simulink model "series_blance_leg"  (R2022b)
settings: Solver=ode45  StartTime=0.0  StopTime=10  MaxStep=0.2  RelTol=1e-3
values from neighbouring files (symbols this model uses):
  a11 = polyfit(leg,k11,3)    [series_get_k.m]
  a12 = polyfit(leg,k12,3)    [series_get_k.m]
  a13 = polyfit(leg,k13,3)    [series_get_k.m]
  a14 = polyfit(leg,k14,3)    [series_get_k.m]
  a15 = polyfit(leg,k15,3)    [series_get_k.m]
  a16 = polyfit(leg,k16,3)    [series_get_k.m]
  a21 = polyfit(leg,k21,3)    [series_get_k.m]
  a22 = polyfit(leg,k22,3)    [series_get_k.m]
  a23 = polyfit(leg,k23,3)    [series_get_k.m]
  a24 = polyfit(leg,k24,3)    [series_get_k.m]
  a25 = polyfit(leg,k25,3)    [series_get_k.m]
  a26 = polyfit(leg,k26,3)    [series_get_k.m]
  N = NM + mp*diff(x + L*sin(theta),t,2)    [series_get_k_length.m]
undefined symbols (not defined in the file or in its folder): X, Y, Z
libraries: sm_lib x60, nesl_utility x20, matrix_library x8, slpidlib x2, cstblocks x2
(part 3 of 3)

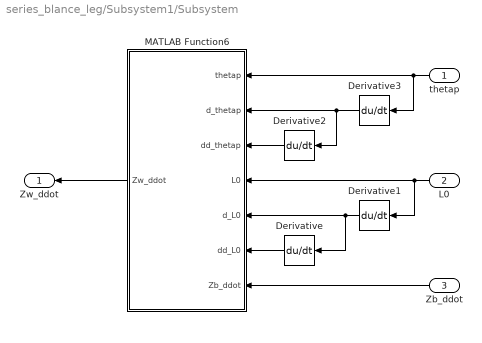
== system series_blance_leg/Subsystem1/Subsystem ==
  thetap : Inport
  L0 : Inport  Port=2
  Zb_ddot : Inport  Port=3
  Derivative{,1..3} (4 alike) : Derivative
  MATLAB Function6 : MATLAB Function  TreatAsAtomicUnit=on
  Zw_ddot : Outport
  wires:
  thetap/1 -> MATLAB Function6/1(thetap), Derivative3/1
  L0/1 -> Derivative1/1, MATLAB Function6/4(L0)
  Derivative1/1 -> Derivative/1, MATLAB Function6/5(d_L0)
  Derivative2/1 -> MATLAB Function6/3(dd_thetap)
  Derivative3/1 -> Derivative2/1, MATLAB Function6/2(d_thetap)
  Derivative/1 -> MATLAB Function6/6(dd_L0)
  Zb_ddot/1 -> MATLAB Function6/7(Zb_ddot)
  MATLAB Function6/1(Zw_ddot) -> Zw_ddot/1

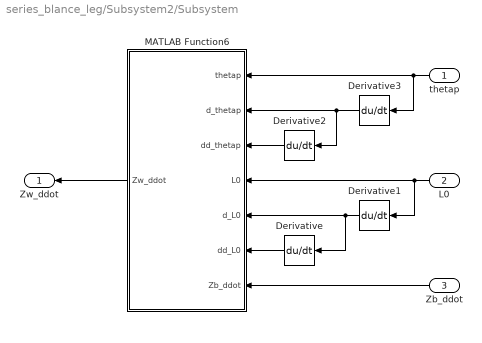
== system series_blance_leg/Subsystem2/Subsystem ==
  thetap : Inport
  L0 : Inport  Port=2
  Zb_ddot : Inport  Port=3
  Derivative{,1..3} (4 alike) : Derivative
  MATLAB Function6 : MATLAB Function  TreatAsAtomicUnit=on
  Zw_ddot : Outport
  wires:
  thetap/1 -> MATLAB Function6/1(thetap), Derivative3/1
  L0/1 -> Derivative1/1, MATLAB Function6/4(L0)
  Derivative1/1 -> Derivative/1, MATLAB Function6/5(d_L0)
  Derivative2/1 -> MATLAB Function6/3(dd_thetap)
  Derivative3/1 -> Derivative2/1, MATLAB Function6/2(d_thetap)
  Derivative/1 -> MATLAB Function6/6(dd_L0)
  Zb_ddot/1 -> MATLAB Function6/7(Zb_ddot)
  MATLAB Function6/1(Zw_ddot) -> Zw_ddot/1

== matlab function series_blance_leg/control/MATLAB Function8 ==
  data: d_phi0 output; theta1 input; theta2 input; d_theta1 input; d_theta2 input
function d_phi0 = D_PHI0(theta1,theta2,d_theta1,d_theta2)
   
    l1=0.3;
    l2=0.3;

    d_phi0 = (d_theta1*l1*(l1 + l2*cos(theta1 - theta2)))/(l1^2 + 2*cos(theta1 - theta2)*l1*l2 + l2^2) + (d_theta2*l2*(l2 + l1*cos(theta1 - theta2)))/(l1^2 + 2*cos(theta1 - theta2)*l1*l2 + l2^2);
 
    
end
    % jacobian函数无法在simulink中使用，故直接使用jacobian函数的最终结果

== matlab function series_blance_leg/calc/MATLAB Function6 ==
  data: k output; a input; length input
function k = get_K(a,length)
   k = polyval(a,length);  
end

== matlab function series_blance_leg/calc/MATLAB Function10 ==
  data: k output; a input; length input
function k = get_K(a,length)
   k = polyval(a,length);  
end

== matlab function series_blance_leg/calc/MATLAB Function11 ==
  data: k output; a input; length input
function k = get_K(a,length)
   k = polyval(a,length);  
end

== matlab function series_blance_leg/calc/MATLAB Function12 ==
  data: k output; a input; length input
function k = get_K(a,length)
   k = polyval(a,length);  
end

== matlab function series_blance_leg/calc/MATLAB Function7 ==
  data: k output; a input; length input
function k = get_K(a,length)
   k = polyval(a,length);  
end

== matlab function series_blance_leg/calc/MATLAB Function8 ==
  data: k output; a input; length input
function k = get_K(a,length)
   k = polyval(a,length);  
end

== matlab function series_blance_leg/control1/MATLAB Function6 ==
  data: F0 input; T1 output; Tp input; theta1 input; theta2 input; T2 output
function [T1,T2] = VMC_calc(F0,Tp,theta1,theta2)
  
l1=0.3;
l2=0.3;
   
j11 = -(l1*l2*sin(theta1 - theta2))/(l1^2 + 2*cos(theta1 - theta2)*l1*l2 + l2^2)^(1/2);
j12 = (l1*l2*sin(theta1 - theta2))/(l1^2 + 2*cos(theta1 - theta2)*l1*l2 + l2^2)^(1/2);
j21 = (l1*(l1 + l2*cos(theta1 - theta2)))/(l1^2 + 2*cos(theta1 - theta2)*l1*l2 + l2^2);
j22 = (l2*(l2 + l1*cos(theta1 - theta2)))/(l1^2 + 2*cos(theta1 - theta2)*l1*l2 + l2^2);
J = [j11 j12; j21 j22];
F = [F0;Tp];
T = J' * F;
T1 = T(1,1);
T2 = T(2,1);

end

== matlab function series_blance_leg/calc/MATLAB Function9 ==
  data: k output; a input; length input
function k = get_K(a,length)
   k = polyval(a,length);  
end

== matlab function series_blance_leg/calc1/MATLAB Function1 ==
  data: k output; a input; length input
function k = get_K(a,length)
   k = polyval(a,length);  
end

== matlab function series_blance_leg/calc1/MATLAB Function10 ==
  data: k output; a input; length input
function k = get_K(a,length)
   k = polyval(a,length);  
end

== matlab function series_blance_leg/calc1/MATLAB Function11 ==
  data: k output; a input; length input
function k = get_K(a,length)
   k = polyval(a,length);  
end

== matlab function series_blance_leg/calc1/MATLAB Function12 ==
  data: k output; a input; length input
function k = get_K(a,length)
   k = polyval(a,length);  
end

== matlab function series_blance_leg/calc1/MATLAB Function2 ==
  data: k output; a input; length input
function k = get_K(a,length)
   k = polyval(a,length);  
end

== matlab function series_blance_leg/calc1/MATLAB Function3 ==
  data: k output; a input; length input
function k = get_K(a,length)
   k = polyval(a,length);  
end

== matlab function series_blance_leg/calc1/MATLAB Function4 ==
  data: k output; a input; length input
function k = get_K(a,length)
   k = polyval(a,length);  
end

== matlab function series_blance_leg/calc1/MATLAB Function5 ==
  data: k output; a input; length input
function k = get_K(a,length)
   k = polyval(a,length);  
end

== matlab function series_blance_leg/calc1/MATLAB Function6 ==
  data: k output; a input; length input
function k = get_K(a,length)
   k = polyval(a,length);  
end

== matlab function series_blance_leg/calc1/MATLAB Function7 ==
  data: k output; a input; length input
function k = get_K(a,length)
   k = polyval(a,length);  
end

== matlab function series_blance_leg/calc1/MATLAB Function8 ==
  data: k output; a input; length input
function k = get_K(a,length)
   k = polyval(a,length);  
end

== matlab function series_blance_leg/calc1/MATLAB Function9 ==
  data: k output; a input; length input
function k = get_K(a,length)
   k = polyval(a,length);  
end

== matlab function series_blance_leg/Subsystem1/MATLAB Function6 ==
  data: thetap input; zw_ddot input; F input; Fn output
function Fn = Fn_calc(thetap,zw_ddot,F)
    
  Mp=5.54; 
  Mw=1.18;
  g=9.8;
  Fn=F*cos(thetap)+Mp*g+Mw*zw_ddot;
end

== matlab function series_blance_leg/control1/MATLAB Function7 ==
  data: L0 output; theta1 input; theta2 input; phi0 output
function [L0,phi0] = L0_PHI0(theta1,theta2)

l1=0.3;
l2=0.3;

xc = l1*cos(theta1) + l2*cos(theta2);
yc = l1*sin(theta1) + l2*sin(theta2);
L0 = sqrt(xc^2+yc^2);
phi0 = atan2(yc,xc);
end

== matlab function series_blance_leg/Subsystem1/Subsystem/MATLAB Function6 ==
  data: thetap input; Zw_ddot output; d_thetap input; dd_thetap input; L0 input; d_L0 input; dd_L0 input; Zb_ddot input
function Zw_ddot = Zw_ddot_calc(thetap,d_thetap,dd_thetap,L0,d_L0,dd_L0,Zb_ddot)

   Zw_ddot=Zb_ddot-dd_L0*cos(thetap)+2*d_L0*d_thetap*sin(thetap)+L0*dd_thetap*sin(thetap)+L0*(d_thetap^2)*cos(thetap);
end

== matlab function series_blance_leg/Subsystem2/MATLAB Function6 ==
  data: thetap input; zw_ddot input; F input; Fn output
function Fn = Fn_calc(thetap,zw_ddot,F)
    
  Mp=5.54; 
  Mw=1.18;
  g=9.8;
  Fn=F*cos(thetap)+Mp*g+Mw*zw_ddot;
end

== matlab function series_blance_leg/Subsystem2/Subsystem/MATLAB Function6 ==
  data: thetap input; Zw_ddot output; d_thetap input; dd_thetap input; L0 input; d_L0 input; dd_L0 input; Zb_ddot input
function Zw_ddot = Zw_ddot_calc(thetap,d_thetap,dd_thetap,L0,d_L0,dd_L0,Zb_ddot)

   Zw_ddot=Zb_ddot-dd_L0*cos(thetap)+2*d_L0*d_thetap*sin(thetap)+L0*dd_thetap*sin(thetap)+L0*(d_thetap^2)*cos(thetap);
end

== matlab function series_blance_leg/calc/MATLAB Function13 ==
  data: k output; a input; length input
function k = get_K(a,length)
   k = polyval(a,length);  
end

== matlab function series_blance_leg/calc/MATLAB Function14 ==
  data: k output; a input; length input
function k = get_K(a,length)
   k = polyval(a,length);  
end

== matlab function series_blance_leg/calc/MATLAB Function15 ==
  data: k output; a input; length input
function k = get_K(a,length)
   k = polyval(a,length);  
end

== matlab function series_blance_leg/calc/MATLAB Function16 ==
  data: k output; a input; length input
function k = get_K(a,length)
   k = polyval(a,length);  
end

== matlab function series_blance_leg/calc/MATLAB Function17 ==
  data: k output; a input; length input
function k = get_K(a,length)
   k = polyval(a,length);  
end

== matlab function series_blance_leg/calc/MATLAB Function18 ==
  data: k output; a input; length input
function k = get_K(a,length)
   k = polyval(a,length);  
end

== matlab function series_blance_leg/control1/MATLAB Function8 ==
  data: d_phi0 output; theta1 input; theta2 input; d_theta1 input; d_theta2 input
function d_phi0 = D_PHI0(theta1,theta2,d_theta1,d_theta2)
   
    l1=0.3;
    l2=0.3;

    d_phi0 = (d_theta1*l1*(l1 + l2*cos(theta1 - theta2)))/(l1^2 + 2*cos(theta1 - theta2)*l1*l2 + l2^2) + (d_theta2*l2*(l2 + l1*cos(theta1 - theta2)))/(l1^2 + 2*cos(theta1 - theta2)*l1*l2 + l2^2);
 
    
end
    % jacobian函数无法在simulink中使用，故直接使用jacobian函数的最终结果

== matlab function series_blance_leg/calc/MATLAB Function19 ==
  data: k output; a input; length input
function k = get_K(a,length)
   k = polyval(a,length);  
end

== matlab function series_blance_leg/calc/MATLAB Function20 ==
  data: k output; a input; length input
function k = get_K(a,length)
   k = polyval(a,length);  
end

== matlab function series_blance_leg/calc/MATLAB Function21 ==
  data: k output; a input; length input
function k = get_K(a,length)
   k = polyval(a,length);  
end

== matlab function series_blance_leg/calc/MATLAB Function22 ==
  data: k output; a input; length input
function k = get_K(a,length)
   k = polyval(a,length);  
end

== matlab function series_blance_leg/calc/MATLAB Function23 ==
  data: k output; a input; length input
function k = get_K(a,length)
   k = polyval(a,length);  
end

== matlab function series_blance_leg/calc/MATLAB Function24 ==
  data: k output; a input; length input
function k = get_K(a,length)
   k = polyval(a,length);  
end

== matlab function series_blance_leg/calc1/MATLAB Function13 ==
  data: k output; a input; length input
function k = get_K(a,length)
   k = polyval(a,length);  
end

== matlab function series_blance_leg/calc1/MATLAB Function14 ==
  data: k output; a input; length input
function k = get_K(a,length)
   k = polyval(a,length);  
end

== matlab function series_blance_leg/calc1/MATLAB Function15 ==
  data: k output; a input; length input
function k = get_K(a,length)
   k = polyval(a,length);  
end

== matlab function series_blance_leg/calc1/MATLAB Function16 ==
  data: k output; a input; length input
function k = get_K(a,length)
   k = polyval(a,length);  
end

== matlab function series_blance_leg/calc1/MATLAB Function17 ==
  data: k output; a input; length input
function k = get_K(a,length)
   k = polyval(a,length);  
end

== matlab function series_blance_leg/calc1/MATLAB Function18 ==
  data: k output; a input; length input
function k = get_K(a,length)
   k = polyval(a,length);  
end

== matlab function series_blance_leg/calc1/MATLAB Function19 ==
  data: k output; a input; length input
function k = get_K(a,length)
   k = polyval(a,length);  
end

== matlab function series_blance_leg/calc/MATLAB Function1 ==
  data: k output; a input; length input
function k = get_K(a,length)
   k = polyval(a,length);  
end

== matlab function series_blance_leg/calc1/MATLAB Function20 ==
  data: k output; a input; length input
function k = get_K(a,length)
   k = polyval(a,length);  
end

== matlab function series_blance_leg/calc1/MATLAB Function21 ==
  data: k output; a input; length input
function k = get_K(a,length)
   k = polyval(a,length);  
end

== matlab function series_blance_leg/calc1/MATLAB Function22 ==
  data: k output; a input; length input
function k = get_K(a,length)
   k = polyval(a,length);  
end

== matlab function series_blance_leg/calc1/MATLAB Function23 ==
  data: k output; a input; length input
function k = get_K(a,length)
   k = polyval(a,length);  
end

== matlab function series_blance_leg/calc1/MATLAB Function24 ==
  data: k output; a input; length input
function k = get_K(a,length)
   k = polyval(a,length);  
end

== matlab function series_blance_leg/calc/MATLAB Function2 ==
  data: k output; a input; length input
function k = get_K(a,length)
   k = polyval(a,length);  
end

== matlab function series_blance_leg/calc/MATLAB Function3 ==
  data: k output; a input; length input
function k = get_K(a,length)
   k = polyval(a,length);  
end

== matlab function series_blance_leg/calc/MATLAB Function4 ==
  data: k output; a input; length input
function k = get_K(a,length)
   k = polyval(a,length);  
end

== matlab function series_blance_leg/calc/MATLAB Function5 ==
  data: k output; a input; length input
function k = get_K(a,length)
   k = polyval(a,length);  
end

== matlab function series_blance_leg/control/MATLAB Function6 ==
  data: F0 input; T1 output; Tp input; theta1 input; theta2 input; T2 output
function [T1,T2] = VMC_calc(F0,Tp,theta1,theta2)
  
l1=0.3;
l2=0.3;
   
j11 = -(l1*l2*sin(theta1 - theta2))/(l1^2 + 2*cos(theta1 - theta2)*l1*l2 + l2^2)^(1/2);
j12 = (l1*l2*sin(theta1 - theta2))/(l1^2 + 2*cos(theta1 - theta2)*l1*l2 + l2^2)^(1/2);
j21 = (l1*(l1 + l2*cos(theta1 - theta2)))/(l1^2 + 2*cos(theta1 - theta2)*l1*l2 + l2^2);
j22 = (l2*(l2 + l1*cos(theta1 - theta2)))/(l1^2 + 2*cos(theta1 - theta2)*l1*l2 + l2^2);
J = [j11 j12; j21 j22];
F = [F0;Tp];
T = J' * F;
T1 = T(1,1);
T2 = T(2,1);

end

== matlab function series_blance_leg/control/MATLAB Function7 ==
  data: L0 output; theta1 input; theta2 input; phi0 output
function [L0,phi0] = L0_PHI0(theta1,theta2)

l1=0.3;
l2=0.3;

xc = l1*cos(theta1) + l2*cos(theta2);
yc = l1*sin(theta1) + l2*sin(theta2);
L0 = sqrt(xc^2+yc^2);
phi0 = atan2(yc,xc);
end
